simulink model "Teleoperation_Config_Space"  (R2021b)
settings: Solver=FixedStepAuto  StartTime=0.0  StopTime=4  FixedStep=Ts  RelTol=1e-3
values from neighbouring files (symbols this model uses):
  alphas_m = 75.0 * ones(1,n)    [setup_teleop.m]
  B_m = diag(ones(1,n)) * 5    [setup_teleop.m]
  B_s = diag(ones(1,n)) * 4    [setup_teleop.m]
  G = 15    [setup_teleop.m]
  gravity = [0 0 9.81]'    [setup_robot.m]
  K_g = eye(n) * k_g    [setup_teleop.m]
  K_m = diag(ones(1,n)) * 10    [setup_teleop.m]
  K_s = diag(ones(1,n)) * 4    [setup_teleop.m]
  lambdas_m = 4.0 * ones(1,n)    [setup_teleop.m]
  M_m = diag(ones(1,n)) * 1    [setup_teleop.m]
  M_s = diag(ones(1,n)) * 1    [setup_teleop.m]
  T_m2s = 0    [setup_teleop.m]
  T_s2m = 0    [setup_teleop.m]
  zdq_A = [1 3*wc 3*wc^2 wc^3]    [setup_teleop.m]
  zdq_B = [0 0 0 wc^3]    [setup_teleop.m]
undefined symbols (not defined in the file or in its folder): alphas_s, conf, dh, Fm_A, Fm_B, Fs_A, Fs_B, lambdas_s, x0
libraries: vrlib x2, simulink x1
settings Model: Creator=eros  LastModifiedBy=Sebastiano
settings SolverCC: AlgebraicLoopSolver=TrustRegion
settings DebuggingCC: SFMachineParentedDataDiag=warning

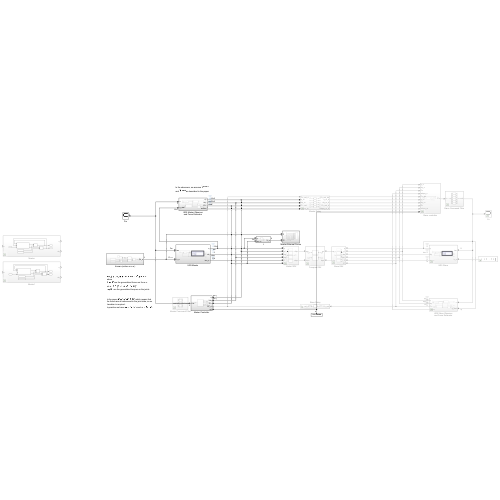
[thumbnail: Simulink's stored preview of the top-level diagram]
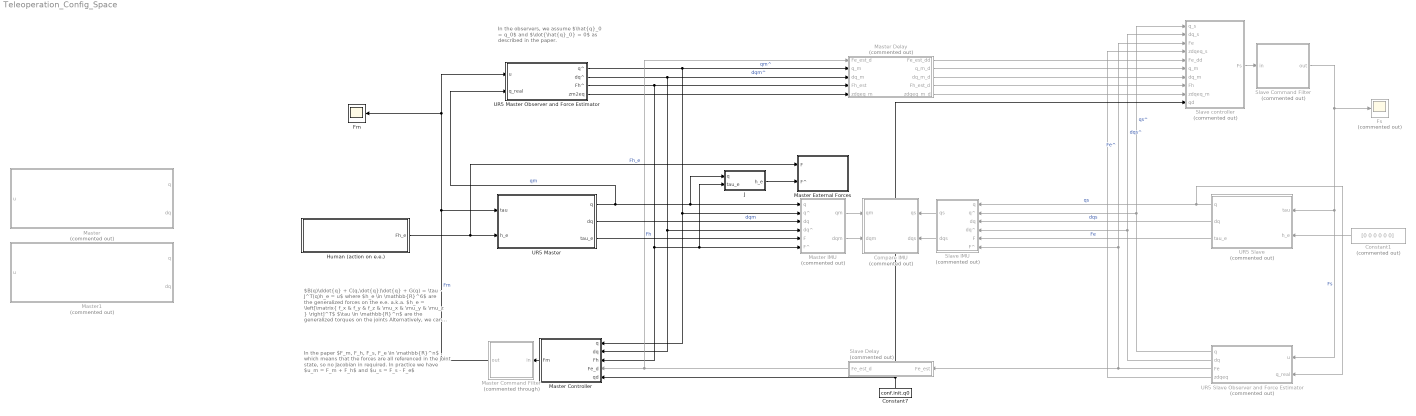
== system Teleoperation_Config_Space ==
  note: In the observers, we assume $\hat{q}_0 = q_0$ and $\dot{\hat{q}_0} = 0$ as described in the paper.
  note: In the paper $F_m, F_h, F_s, F_e \in \mathbb{R}^n$ , which means that the forces are all referenced in the joint state, so no Jacobian in required.
      | In practice we have $u_m = F_m + F_h$ and $u_s = F_s - F_e$
  note: $B(q)\ddot{q} + C(q,\dot{q})\dot{q} + G(q) = \tau - J^T(q)h_e = u$
      | where
      | $h_e \in \mathbb{R}^6$ are the generalized forces on the e.e.
      | a.k.a. $h_e = \left[\matrix{ f_x & f_y & f_z & \mu_x & \mu_y & \mu_z } \right]^T$
      | $\tau \in \mathbb{R}^n$ are the generalized torques on the joints
      |
      | Alternatively, we can write $\tau = J^T(q)\tau_e$ .
  Compare IMU : Subsystem  Commented=on
      settings: PortSchema="{\"entries\":[{\"content\":{\"sides\":[{\"content\":{\"connectorIds\":[\"In1\",\"In2\"]},\"type\":\"ConnectorPlacement.EquallySpacedRectSide\",\"uuid\":\"eee4eb85-6cb8-4462-85fc-1aafb3c3937f\"},{\"content\":{\"connectorIds\":[\"In3\",\"In4\"],\"side\":\"RIGHT\"},\"type\":\"ConnectorPlacement.EquallySpacedRectSide\",\"uuid\":\"5ab37ec6-6ee1-47e9-aff6-41baaee9b59b\"},{\"content\":{\"connectorIds\":[],\"side\":\"TOP\"},\"type\":\"ConnectorPlacement.EquallySpacedRectSide\",\"uuid\":\"6f11ee79-2d90-4b50-8360-b99d360f33b3\"}]},\"type\":\"ConnectorPlacement.EquallySpacedConnector\",\"uuid\":\"5676dc65-12f4-4a54-a0ce-a07c6c462ad2\"}],\"packageUris\":[\"http://schema.mathworks.com/mf0/Connector/R2020b\"],\"version\":\"1.0\"}"
  Constant1 : Constant  Commented=on  Value=[0 0 0 0 0 0]
  Constant7 : Constant  Value=conf.init.q0
  Fm : Scope
  Fs : Scope  Commented=on
  Human (action on e.e.) : Subsystem
  J : Subsystem
  Master : Subsystem  Commented=on
  Master Command Filter : Subsystem  Commented=through
  Master Controller : Subsystem
  Master Delay : Subsystem  Commented=on
  Master External Forces : Subsystem
  Master IMU : Subsystem  Commented=on
  Master1 : Subsystem  Commented=on
  Slave Command Filter : Subsystem  Commented=on
  Slave Delay : Subsystem  Commented=on
  Slave IMU : Subsystem  Commented=on
  Slave controller : Subsystem  Commented=on
  UR5 Master : Subsystem
  UR5 Master Observer and Force Estimator : Subsystem
  UR5 Slave : Subsystem  Commented=on
  UR5 Slave Observer and Force Estimator : Subsystem  Commented=on
  wires:
  UR5 Slave Observer and Force Estimator/1(q) -> Slave IMU/2(q^), Slave controller/1(q_s)  "qs^"
  Master Controller/1(Fm) -> Master Command Filter/1(in)
  UR5 Slave Observer and Force Estimator/4(zdqeq) -> Slave controller/4(zdqeq_s)
  UR5 Master Observer and Force Estimator/1(q^) -> Master Controller/1(q), Master IMU/2(q^), Master Delay/2(q_m)  "qm^"
  UR5 Slave Observer and Force Estimator/3(Fe) -> Slave controller/3(Fe), Slave IMU/6(F^), Slave Delay/1(Fe_est)  "Fe^"
  UR5 Master Observer and Force Estimator/3(Fh^) -> Master IMU/6(F^), J/2(tau_e), Master Controller/3(Fh), Master Delay/4(Fh_est)
  UR5 Slave Observer and Force Estimator/2(dq) -> Slave IMU/4(dq^), Slave controller/2(dq_s)  "dqs^"
  UR5 Master Observer and Force Estimator/2(dq^) -> Master Controller/2(dq), Master IMU/4(dq^), Master Delay/3(dq_m)  "dqm^"
  Slave controller/1(Fs) -> Slave Command Filter/1(in)
  Master Command Filter/1(out) -> UR5 Master Observer and Force Estimator/1(u), Fm/1, UR5 Master/1(tau)  "Fm"
  Slave Command Filter/1(out) -> UR5 Slave/1(tau), UR5 Slave Observer and Force Estimator/1(u), Fs/1  "Fs"
  UR5 Master Observer and Force Estimator/4(zm2eq) -> Master Delay/5(zdqeq_m)
  Master Delay/1(Fe_est_dd) -> Slave controller/5(Fe_dd)
  Master Delay/3(dq_m_d) -> Slave controller/7(dq_m)
  Master Delay/2(q_m_d) -> Slave controller/6(q_m)
  Master Delay/4(Fh_est_d) -> Slave controller/8(Fh)
  Master Delay/5(zdqeq_m_d) -> Slave controller/9(zdqeq_m)
  Slave Delay/1(Fe_est_d) -> Master Delay/1(Fe_est_d), Master Controller/4(Fe_d)
  UR5 Slave/1(q) -> UR5 Slave Observer and Force Estimator/2(q_real), Slave IMU/1(q)  "qs"
  UR5 Slave/2(dq) -> Slave IMU/3(dq)  "dqs"
  Constant1/1 -> UR5 Slave/2(h_e)
  UR5 Slave/3(tau_e) -> Slave IMU/5(F)  "Fe"
  Constant7/1 -> Master Controller/5(qd), Slave controller/10(qd)
  J/1(h_e) -> Master External Forces/2(F^)
  Human (action on e.e.)/1(Fh_e) -> Master External Forces/1(F), UR5 Master/2(h_e)  "Fh_e"
  UR5 Master/1(q) -> UR5 Master Observer and Force Estimator/2(q_real), J/1(q), Master IMU/1(q)  "qm"
  UR5 Master/2(dq) -> Master IMU/3(dq)  "dqm"
  UR5 Master/3(tau_e) -> Master IMU/5(F)  "Fh"
  Master IMU/1(qm) -> Compare IMU/1(qm)
  Master IMU/2(dqm) -> Compare IMU/2(dqm)
  Slave IMU/1(qs) -> Compare IMU/3(qs)
  Slave IMU/2(dqs) -> Compare IMU/4(dqs)

== system Teleoperation_Config_Space/Compare IMU ==
  qm : Inport
  dqm : Inport  Port=2
  qs : Inport  Port=3
  dqs : Inport  Port=4
  State : Subsystem
      settings: PortSchema="{\"entries\":[{\"content\":{\"sides\":[{\"content\":{\"connectorIds\":[\"In1\"]},\"type\":\"ConnectorPlacement.EquallySpacedRectSide\",\"uuid\":\"98f8c5d8-e26e-427c-a81e-60bbe3a3ab4d\"},{\"content\":{\"connectorIds\":[\"In2\"],\"side\":\"RIGHT\"},\"type\":\"ConnectorPlacement.EquallySpacedRectSide\",\"uuid\":\"a51aa647-09cd-4fb3-b31a-f2bc2bc6e0ff\"},{\"content\":{\"connectorIds\":[],\"side\":\"TOP\"},\"type\":\"ConnectorPlacement.EquallySpacedRectSide\",\"uuid\":\"9387bbe5-2fda-43cb-b346-55f243092f42\"}]},\"type\":\"ConnectorPlacement.EquallySpacedConnector\",\"uuid\":\"8debe184-3b59-4f16-84f4-2d6030e17ba5\"}],\"packageUris\":[\"http://schema.mathworks.com/mf0/Connector/R2020b\"],\"version\":\"1.0\"}"
  Velocity : Subsystem
      settings: PortSchema="{\"entries\":[{\"content\":{\"sides\":[{\"content\":{\"connectorIds\":[\"In1\"]},\"type\":\"ConnectorPlacement.EquallySpacedRectSide\",\"uuid\":\"98f8c5d8-e26e-427c-a81e-60bbe3a3ab4d\"},{\"content\":{\"connectorIds\":[\"In2\"],\"side\":\"RIGHT\"},\"type\":\"ConnectorPlacement.EquallySpacedRectSide\",\"uuid\":\"a51aa647-09cd-4fb3-b31a-f2bc2bc6e0ff\"},{\"content\":{\"connectorIds\":[],\"side\":\"TOP\"},\"type\":\"ConnectorPlacement.EquallySpacedRectSide\",\"uuid\":\"9387bbe5-2fda-43cb-b346-55f243092f42\"}]},\"type\":\"ConnectorPlacement.EquallySpacedConnector\",\"uuid\":\"8debe184-3b59-4f16-84f4-2d6030e17ba5\"}],\"packageUris\":[\"http://schema.mathworks.com/mf0/Connector/R2020b\"],\"version\":\"1.0\"}"
  wires:
  qm/1 -> State/2(q_m)
  qs/1 -> State/1(q_s)
  dqm/1 -> Velocity/1(dq_m)
  dqs/1 -> Velocity/2(dq_s)

== system Teleoperation_Config_Space/Human (action on e.e.) ==
  Constant2 : Constant  Value=[0 1 0 0 0 0]
  Constant4 : Constant  Value=[0 0 1 0 0 0]
  Manual Switch : ManualSwitch  CurrentSetting=0
  Matrix Multiply : Product
  Multiply : Gain  Gain=G
  Pulse Generator : DiscretePulseGenerator  PulseType=Time based  TimeSource=Use external signal  Period=1.5  PulseWidth=50  PhaseDelay=0.5
  Switch : Switch  Criteria=u2 > Threshold  Threshold=1.75
  Time : simulink/Sources/Ramp  slope=1  start=0  InitialOutput=0
  Transfer Fcn : TransferFcn  Numerator=[2*pi*5]  Denominator=[1 2*pi*5]
  Fh_e : Outport
  wires:
  Pulse Generator/1 -> Multiply/1
  Switch/1 -> Matrix Multiply/2
  Constant2/1 -> Manual Switch/2
  Transfer Fcn/1 -> Matrix Multiply/1
  Time/1 -> Switch/2, Pulse Generator/1
  Constant4/1 -> Manual Switch/1, Switch/1
  Matrix Multiply/1 -> Fh_e/1
  Multiply/1 -> Transfer Fcn/1
  Manual Switch/1 -> Switch/3

== system Teleoperation_Config_Space/J ==
  q : Inport
  tau_e : Inport  Port=2
  MATLAB Function : MATLAB Function  TreatAsAtomicUnit=on
  Matrix Multiply : Product  Multiplication=Matrix(*)
  h_e : Outport
  wires:
  MATLAB Function/1(J) -> Matrix Multiply/1
  Matrix Multiply/1 -> h_e/1
  tau_e/1 -> Matrix Multiply/2
  q/1 -> MATLAB Function/1(q)

== system Teleoperation_Config_Space/Master ==
  u : Inport
  Constant : Constant  Value=conf.init.q0
  Constant1 : Constant  Value=conf.init.dq0
  Integrator : Integrator  InitialConditionSource=external
  Integrator1 : Integrator  InitialConditionSource=external
  MATLAB Function : MATLAB Function  TreatAsAtomicUnit=on
  q : Outport
  dq : Outport  Port=2
  wires:
  MATLAB Function/1(dq) -> Integrator/1
  MATLAB Function/2(ddq) -> Integrator1/1
  Integrator/1 -> MATLAB Function/1(q), q/1
  Integrator1/1 -> MATLAB Function/2("dq "), dq/1
  u/1 -> MATLAB Function/3(u)
  Constant/1 -> Integrator/2
  Constant1/1 -> Integrator1/2

== system Teleoperation_Config_Space/Master Command Filter ==
  in : Inport
  Demux : Demux  Outputs=6
  Filter{,1..5} (6 alike) : TransferFcn  Numerator=Fm_B  Denominator=Fm_A
  Mux : Mux  Inputs=6
  out : Outport
  wires:
  Demux/4 -> Filter3/1
  Demux/6 -> Filter5/1
  Demux/2 -> Filter1/1
  Demux/5 -> Filter4/1
  Demux/1 -> Filter/1
  Demux/3 -> Filter2/1
  in/1 -> Demux/1
  Mux/1 -> out/1
  Filter/1 -> Mux/1
  Filter1/1 -> Mux/2
  Filter2/1 -> Mux/3
  Filter3/1 -> Mux/4
  Filter4/1 -> Mux/5
  Filter5/1 -> Mux/6

== system Teleoperation_Config_Space/Master Controller ==
  q : Inport
  dq : Inport  Port=2
  Fh : Inport  Port=3
  Fe_d : Inport  Port=4
  qd : Inport  Port=5
  Master Controller : MATLAB Function  TreatAsAtomicUnit=on
  Fm : Outport
  wires:
  Fh/1 -> Master Controller/3(Fh)
  Fe_d/1 -> Master Controller/4(Fe_d)
  Master Controller/1(Fm) -> Fm/1  "Fm"
  q/1 -> Master Controller/1(q)
  dq/1 -> Master Controller/2(dq)
  qd/1 -> Master Controller/5(qd)

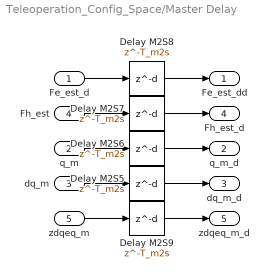
== system Teleoperation_Config_Space/Master Delay ==
  Fe_est_d : Inport
  q_m : Inport  Port=2
  dq_m : Inport  Port=3
  Fh_est : Inport  Port=4
  zdqeq_m : Inport  Port=5
  Delay M2S{5..9} (5 alike) : Delay  DelayLength=T_m2s
  Fe_est_dd : Outport
  q_m_d : Outport  Port=2
  dq_m_d : Outport  Port=3
  Fh_est_d : Outport  Port=4
  zdqeq_m_d : Outport  Port=5
  wires:
  zdqeq_m/1 -> Delay M2S9/1
  Delay M2S6/1 -> q_m_d/1
  dq_m/1 -> Delay M2S5/1
  Fe_est_d/1 -> Delay M2S8/1
  Fh_est/1 -> Delay M2S7/1
  Delay M2S5/1 -> dq_m_d/1
  Delay M2S7/1 -> Fh_est_d/1
  q_m/1 -> Delay M2S6/1
  Delay M2S8/1 -> Fe_est_dd/1
  Delay M2S9/1 -> zdqeq_m_d/1

== system Teleoperation_Config_Space/Master External Forces ==
  F : Inport
  F^ : Inport  Port=2
  Master he : Scope  NumInputPorts=6
  Mux{,1..2,4..6} (6 alike) : Mux  Inputs=2
  qm : Demux  Outputs=dh.dof
  qs : Demux  Outputs=dh.dof
  wires:
  F/1 -> qm/1
  F^/1 -> qs/1
  qm/1 -> Mux/1
  qs/1 -> Mux/2
  qm/2 -> Mux1/1
  qs/2 -> Mux1/2
  qm/3 -> Mux2/1
  qs/3 -> Mux2/2
  qm/4 -> Mux4/1
  qs/4 -> Mux4/2
  Mux/1 -> Master he/1
  Mux1/1 -> Master he/2
  Mux2/1 -> Master he/3
  Mux4/1 -> Master he/4
  Mux5/1 -> Master he/5
  Mux6/1 -> Master he/6
  qs/5 -> Mux5/2
  qm/5 -> Mux5/1
  qm/6 -> Mux6/1
  qs/6 -> Mux6/2

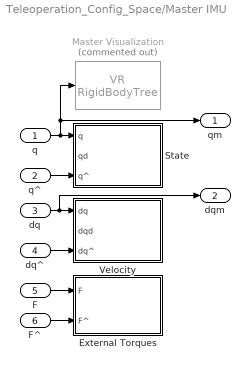
== system Teleoperation_Config_Space/Master IMU ==
  q : Inport
  q^ : Inport  Port=2
  dq : Inport  Port=3
  dq^ : Inport  Port=4
  F : Inport  Port=5
  F^ : Inport  Port=6
  External Torques : Subsystem
  Master Visualization : vrlib/VR RigidBodyTree  Commented=on  RBT=UR5_robot  useRBT=on  Ts=-1  ForceViewerOpen=on
      settings: SourceProductBaseCode=SL
  State : Subsystem
  Velocity : Subsystem
  qm : Outport
  dqm : Outport  Port=2
  wires:
  q/1 -> Master Visualization/1, qm/1, State/1(q)
  q^/1 -> State/3(q^)
  dq/1 -> dqm/1, Velocity/1(dq)
  dq^/1 -> Velocity/3(dq^)
  F/1 -> External Torques/1(F)
  F^/1 -> External Torques/2(F^)

== system Teleoperation_Config_Space/Master1 ==
  u : Inport
  Constant : Constant  Value=conf.init.q0
  Constant1 : Constant  Value=conf.init.dq0
  Integrator : Integrator  InitialConditionSource=external
  Integrator1 : Integrator  InitialConditionSource=external
  MATLAB Function : MATLAB Function  TreatAsAtomicUnit=on
  q : Outport
  dq : Outport  Port=2
  wires:
  MATLAB Function/1(dX) -> Integrator/1
  MATLAB Function/2(ddX) -> Integrator1/1
  Integrator/1 -> q/1, MATLAB Function/1(X)
  Integrator1/1 -> MATLAB Function/2("dX "), dq/1
  u/1 -> MATLAB Function/4(u)
  Constant/1 -> Integrator/2
  Constant1/1 -> Integrator1/2

== system Teleoperation_Config_Space/Slave Command Filter ==
  in : Inport
  Demux : Demux  Outputs=6
  Filter{,1..5} (6 alike) : TransferFcn  Numerator=Fs_B  Denominator=Fs_A
  Mux : Mux  Inputs=6
  out : Outport
  wires:
  Demux/4 -> Filter3/1
  Demux/6 -> Filter5/1
  Demux/2 -> Filter1/1
  Demux/5 -> Filter4/1
  Demux/1 -> Filter/1
  Demux/3 -> Filter2/1
  in/1 -> Demux/1
  Mux/1 -> out/1
  Filter/1 -> Mux/1
  Filter2/1 -> Mux/3
  Filter3/1 -> Mux/4
  Filter4/1 -> Mux/5
  Filter5/1 -> Mux/6
  Filter1/1 -> Mux/2

== system Teleoperation_Config_Space/Slave Delay ==
  Fe_est : Inport
  Delay S2M1 : Delay  DelayLength=T_s2m
  Fe_est_d : Outport
  wires:
  Delay S2M1/1 -> Fe_est_d/1
  Fe_est/1 -> Delay S2M1/1

== system Teleoperation_Config_Space/Slave IMU ==
  q : Inport
  q^ : Inport  Port=2
  dq : Inport  Port=3
  dq^ : Inport  Port=4
  F : Inport  Port=5
  F^ : Inport  Port=6
  External Forces : Subsystem
  Master Visualization : vrlib/VR RigidBodyTree  Commented=on  RBT=UR5_robot  useRBT=on  Ts=-1  ForceViewerOpen=on
      settings: SourceProductBaseCode=SL
  State : Subsystem
  Velocity : Subsystem
  qs : Outport
  dqs : Outport  Port=2
  wires:
  q/1 -> Master Visualization/1, qs/1, State/1(q)
  q^/1 -> State/3(q^)
  F/1 -> External Forces/1(F)
  dq/1 -> dqs/1, Velocity/1(dq)
  F^/1 -> External Forces/2(F^)
  dq^/1 -> Velocity/3(dq^)

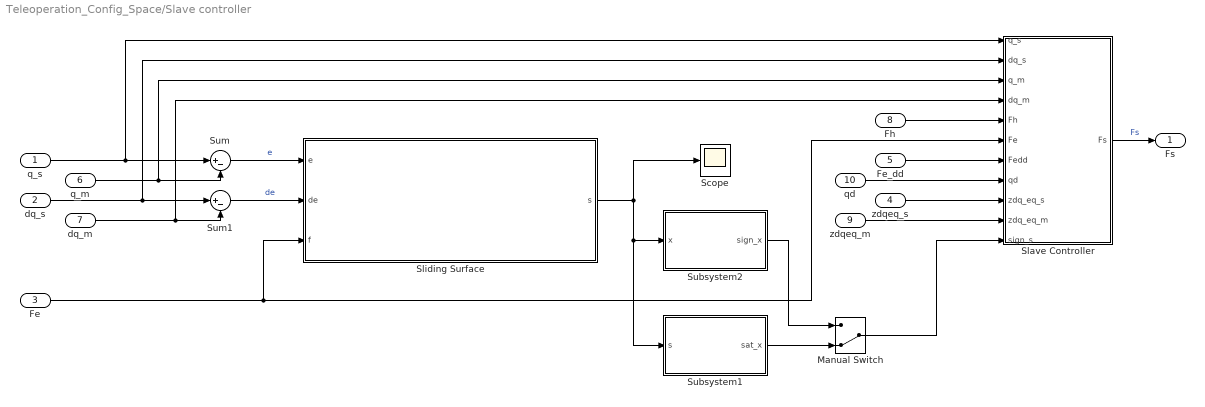
== system Teleoperation_Config_Space/Slave controller ==
  q_s : Inport
  dq_s : Inport  Port=2
  Fe : Inport  Port=3
  zdqeq_s : Inport  Port=4
  Fe_dd : Inport  Port=5
  q_m : Inport  Port=6
  dq_m : Inport  Port=7
  Fh : Inport  Port=8
  zdqeq_m : Inport  Port=9
  qd : Inport  Port=10
  Manual Switch : ManualSwitch  CurrentSetting=0
  Scope : Scope
  Slave Controller : MATLAB Function  TreatAsAtomicUnit=on
  Sliding Surface : Subsystem
  Subsystem1 : Subsystem
  Subsystem2 : Subsystem
  Sum : Sum  Inputs=|+-
  Sum1 : Sum  Inputs=|+-
  Fs : Outport
  wires:
  zdqeq_s/1 -> Slave Controller/9(zdq_eq_s)
  Fh/1 -> Slave Controller/5(Fh)
  Slave Controller/1(Fs) -> Fs/1  "Fs"
  zdqeq_m/1 -> Slave Controller/10(zdq_eq_m)
  Fe_dd/1 -> Slave Controller/7(Fedd)
  q_s/1 -> Sum/1, Slave Controller/1(q_s)
  q_m/1 -> Sum/2, Slave Controller/3(q_m)
  dq_s/1 -> Sum1/1, Slave Controller/2(dq_s)
  dq_m/1 -> Slave Controller/4(dq_m), Sum1/2
  Fe/1 -> Slave Controller/6(Fe), Sliding Surface/3(f)
  Subsystem2/1(sign_x) -> Manual Switch/1
  Sum/1 -> Sliding Surface/1(e)  "e"
  Sum1/1 -> Sliding Surface/2(de)  "de"
  Sliding Surface/1(s) -> Scope/1, Subsystem1/1(s), Subsystem2/1(x)
  qd/1 -> Slave Controller/8(qd)
  Subsystem1/1(sat_x) -> Manual Switch/2
  Manual Switch/1 -> Slave Controller/11(sign_s)

== system Teleoperation_Config_Space/UR5 Master ==
  note: UR5
  tau : Inport
  h_e : Inport  Port=2
  Constant2 : Constant  Value=conf.init.dq0
  Constant6 : Constant  Value=gravity
  Constant7 : Constant  Value=conf.init.q0
  JT : Subsystem
  Robot Model : Subsystem
  Sum4 : Sum  Inputs=++|
  q : Outport
  dq : Outport  Port=2
  tau_e : Outport  Port=3
  wires:
  Robot Model/1(dq) -> dq/1
  tau/1 -> Sum4/1
  Robot Model/2(q) -> JT/2(q), q/1
  JT/1(tau_e) -> tau_e/1, Sum4/2
  h_e/1 -> JT/1(h_e)
  Constant7/1 -> Robot Model/4(q0)
  Constant2/1 -> Robot Model/3(dq0)
  Constant6/1 -> Robot Model/2(g)
  Sum4/1 -> Robot Model/1(u)

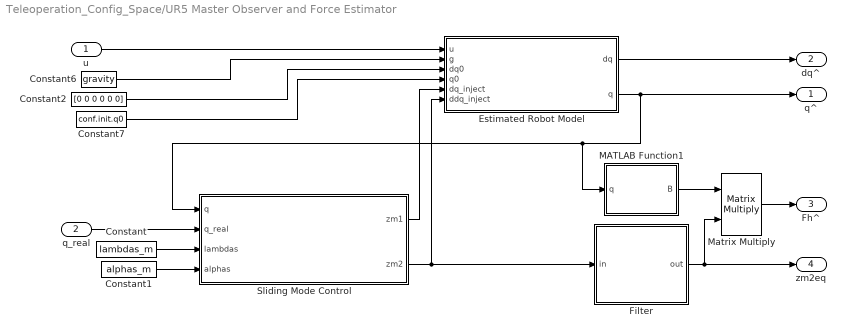
== system Teleoperation_Config_Space/UR5 Master Observer and Force Estimator ==
  u : Inport
  q_real : Inport  Port=2
  Constant : Constant  Value=lambdas_m
  Constant1 : Constant  Value=alphas_m
  Constant2 : Constant  Value=[0 0 0 0 0 0]
  Constant6 : Constant  Value=gravity
  Constant7 : Constant  Value=conf.init.q0
  Estimated Robot Model : Subsystem
  Filter : Subsystem
  MATLAB Function1 : MATLAB Function  TreatAsAtomicUnit=on
  Matrix Multiply : Product  Multiplication=Matrix(*)
  Sliding Mode Control : Subsystem
  q^ : Outport
  dq^ : Outport  Port=2
  Fh^ : Outport  Port=3
  zm2eq : Outport  Port=4
  wires:
  Matrix Multiply/1 -> Fh^/1
  Filter/1(out) -> zm2eq/1, Matrix Multiply/2
  Sliding Mode Control/1(zm1) -> Estimated Robot Model/5(dq_inject)
  Constant7/1 -> Estimated Robot Model/4(q0)
  Constant2/1 -> Estimated Robot Model/3(dq0)
  Constant6/1 -> Estimated Robot Model/2(g)
  u/1 -> Estimated Robot Model/1(u)
  Sliding Mode Control/2(zm2) -> Estimated Robot Model/6(ddq_inject), Filter/1(in)
  MATLAB Function1/1(B) -> Matrix Multiply/1
  Constant1/1 -> Sliding Mode Control/4(alphas)
  Constant/1 -> Sliding Mode Control/3(lambdas)
  q_real/1 -> Sliding Mode Control/2(q_real)
  Estimated Robot Model/2(q) -> q^/1, MATLAB Function1/1(q), Sliding Mode Control/1(q)
  Estimated Robot Model/1(dq) -> dq^/1

== system Teleoperation_Config_Space/UR5 Slave ==
  note: UR5
  tau : Inport
  h_e : Inport  Port=2
  Constant2 : Constant  Value=conf.init.dq0
  Constant6 : Constant  Value=gravity
  Constant7 : Constant  Value=conf.init.q0
  JT : Subsystem
  Robot Model : Subsystem
  Sum4 : Sum  Inputs=+-|
  q : Outport
  dq : Outport  Port=2
  tau_e : Outport  Port=3
  wires:
  Robot Model/1(dq) -> dq/1
  tau/1 -> Sum4/1
  Robot Model/2(q) -> JT/2(q), q/1
  JT/1(tau_e) -> tau_e/1, Sum4/2
  h_e/1 -> JT/1(h_e)
  Constant7/1 -> Robot Model/4(q0)
  Constant2/1 -> Robot Model/3(dq0)
  Constant6/1 -> Robot Model/2(g)
  Sum4/1 -> Robot Model/1(u)

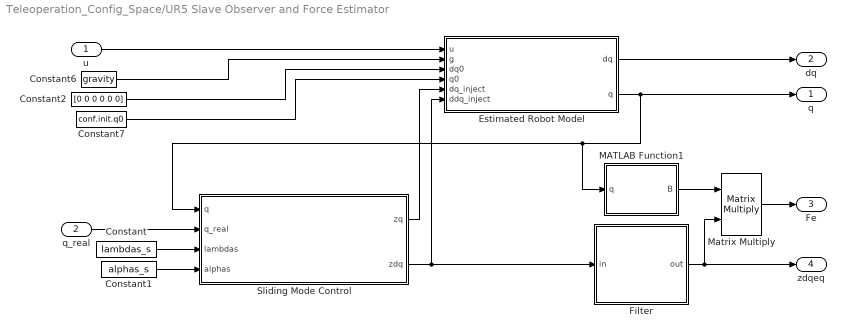
== system Teleoperation_Config_Space/UR5 Slave Observer and Force Estimator ==
  u : Inport
  q_real : Inport  Port=2
  Constant : Constant  Value=lambdas_s
  Constant1 : Constant  Value=alphas_s
  Constant2 : Constant  Value=[0 0 0 0 0 0]
  Constant6 : Constant  Value=gravity
  Constant7 : Constant  Value=conf.init.q0
  Estimated Robot Model : Subsystem
  Filter : Subsystem
  MATLAB Function1 : MATLAB Function  TreatAsAtomicUnit=on
  Matrix Multiply : Product  Multiplication=Matrix(*)
  Sliding Mode Control : Subsystem
  q : Outport
  dq : Outport  Port=2
  Fe : Outport  Port=3
  zdqeq : Outport  Port=4
  wires:
  Estimated Robot Model/2(q) -> MATLAB Function1/1(q), Sliding Mode Control/1(q), q/1
  Estimated Robot Model/1(dq) -> dq/1
  Matrix Multiply/1 -> Fe/1
  Filter/1(out) -> zdqeq/1, Matrix Multiply/2
  Sliding Mode Control/1(zq) -> Estimated Robot Model/5(dq_inject)
  Constant7/1 -> Estimated Robot Model/4(q0)
  Constant2/1 -> Estimated Robot Model/3(dq0)
  Constant6/1 -> Estimated Robot Model/2(g)
  u/1 -> Estimated Robot Model/1(u)
  Sliding Mode Control/2(zdq) -> Filter/1(in), Estimated Robot Model/6(ddq_inject)
  MATLAB Function1/1(B) -> Matrix Multiply/1
  Constant1/1 -> Sliding Mode Control/4(alphas)
  Constant/1 -> Sliding Mode Control/3(lambdas)
  q_real/1 -> Sliding Mode Control/2(q_real)

== system Teleoperation_Config_Space/Compare IMU/State ==
  q_s : Inport
  q_m : Inport  Port=2
  Compare State : Scope  NumInputPorts=6
  Mux{,1..2,4..6} (6 alike) : Mux  Inputs=2
  qm : Demux  Outputs=dh.dof
  qs : Demux  Outputs=dh.dof
  wires:
  q_m/1 -> qm/1
  q_s/1 -> qs/1
  qm/1 -> Mux/1
  qs/1 -> Mux/2
  qm/2 -> Mux1/1
  qs/2 -> Mux1/2
  qm/3 -> Mux2/1
  qs/3 -> Mux2/2
  qm/4 -> Mux4/1
  qs/4 -> Mux4/2
  Mux/1 -> Compare State/1
  Mux1/1 -> Compare State/2
  Mux2/1 -> Compare State/3
  Mux4/1 -> Compare State/4
  Mux5/1 -> Compare State/5
  Mux6/1 -> Compare State/6
  qs/5 -> Mux5/2
  qm/5 -> Mux5/1
  qm/6 -> Mux6/1
  qs/6 -> Mux6/2

== system Teleoperation_Config_Space/Compare IMU/Velocity ==
  dq_m : Inport
  dq_s : Inport  Port=2
  Compare Speed : Scope  NumInputPorts=6
  Mux{,1..2,4..6} (6 alike) : Mux  Inputs=2
  qm : Demux  Outputs=dh.dof
  qs : Demux  Outputs=dh.dof
  wires:
  dq_m/1 -> qm/1
  dq_s/1 -> qs/1
  qm/1 -> Mux/1
  qs/1 -> Mux/2
  qm/2 -> Mux1/1
  qs/2 -> Mux1/2
  qm/3 -> Mux2/1
  qs/3 -> Mux2/2
  qm/4 -> Mux4/1
  qs/4 -> Mux4/2
  Mux/1 -> Compare Speed/1
  Mux1/1 -> Compare Speed/2
  Mux2/1 -> Compare Speed/3
  Mux4/1 -> Compare Speed/4
  Mux5/1 -> Compare Speed/5
  Mux6/1 -> Compare Speed/6
  qs/5 -> Mux5/2
  qm/5 -> Mux5/1
  qm/6 -> Mux6/1
  qs/6 -> Mux6/2

== system Teleoperation_Config_Space/Master IMU/External Torques ==
  F : Inport
  F^ : Inport  Port=2
  Master Fh : Scope  NumInputPorts=6
  Mux{,1..2,4..6} (6 alike) : Mux  Inputs=2
  qm : Demux  Outputs=dh.dof
  qs : Demux  Outputs=dh.dof
  wires:
  F/1 -> qm/1
  F^/1 -> qs/1
  qm/1 -> Mux/1
  qs/1 -> Mux/2
  qm/2 -> Mux1/1
  qs/2 -> Mux1/2
  qm/3 -> Mux2/1
  qs/3 -> Mux2/2
  qm/4 -> Mux4/1
  qs/4 -> Mux4/2
  Mux/1 -> Master Fh/1
  Mux1/1 -> Master Fh/2
  Mux2/1 -> Master Fh/3
  Mux4/1 -> Master Fh/4
  Mux5/1 -> Master Fh/5
  Mux6/1 -> Master Fh/6
  qs/5 -> Mux5/2
  qm/5 -> Mux5/1
  qm/6 -> Mux6/1
  qs/6 -> Mux6/2

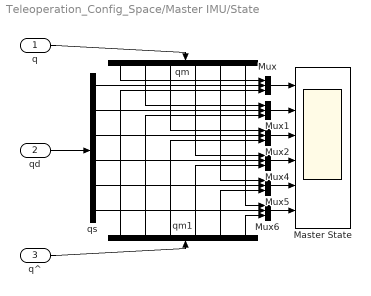
== system Teleoperation_Config_Space/Master IMU/State ==
  q : Inport
  qd : Inport  Port=2
  q^ : Inport  Port=3
  Master State : Scope  NumInputPorts=6
  Mux{,1..2,4..6} (6 alike) : Mux  Inputs=3
  qm : Demux  Outputs=dh.dof
  qm1 : Demux  Outputs=dh.dof
  qs : Demux  Outputs=dh.dof
  wires:
  q/1 -> qm/1
  qd/1 -> qs/1
  qm/1 -> Mux/1
  qs/1 -> Mux/2
  qm/2 -> Mux1/1
  qs/2 -> Mux1/2
  qm/3 -> Mux2/1
  qs/3 -> Mux2/2
  qm/4 -> Mux4/1
  qs/4 -> Mux4/2
  Mux/1 -> Master State/1
  Mux1/1 -> Master State/2
  Mux2/1 -> Master State/3
  Mux4/1 -> Master State/4
  Mux5/1 -> Master State/5
  Mux6/1 -> Master State/6
  qs/5 -> Mux5/2
  qm/5 -> Mux5/1
  qm/6 -> Mux6/1
  qs/6 -> Mux6/2
  qm1/3 -> Mux2/3
  qm1/2 -> Mux1/3
  qm1/4 -> Mux4/3
  qm1/5 -> Mux5/3
  q^/1 -> qm1/1
  qm1/1 -> Mux/3
  qm1/6 -> Mux6/3

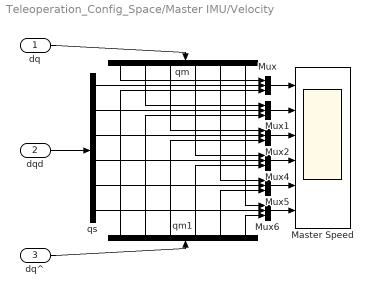
== system Teleoperation_Config_Space/Master IMU/Velocity ==
  dq : Inport
  dqd : Inport  Port=2
  dq^ : Inport  Port=3
  Master Speed : Scope  NumInputPorts=6
  Mux{,1..2,4..6} (6 alike) : Mux  Inputs=3
  qm : Demux  Outputs=dh.dof
  qm1 : Demux  Outputs=dh.dof
  qs : Demux  Outputs=dh.dof
  wires:
  dq/1 -> qm/1
  dqd/1 -> qs/1
  qm/1 -> Mux/1
  qs/1 -> Mux/2
  qm/2 -> Mux1/1
  qs/2 -> Mux1/2
  qm/3 -> Mux2/1
  qs/3 -> Mux2/2
  qm/4 -> Mux4/1
  qs/4 -> Mux4/2
  Mux/1 -> Master Speed/1
  Mux1/1 -> Master Speed/2
  Mux2/1 -> Master Speed/3
  Mux4/1 -> Master Speed/4
  Mux5/1 -> Master Speed/5
  Mux6/1 -> Master Speed/6
  qs/5 -> Mux5/2
  qm/5 -> Mux5/1
  qm/6 -> Mux6/1
  qs/6 -> Mux6/2
  qm1/3 -> Mux2/3
  qm1/2 -> Mux1/3
  qm1/4 -> Mux4/3
  qm1/5 -> Mux5/3
  dq^/1 -> qm1/1
  qm1/1 -> Mux/3
  qm1/6 -> Mux6/3

== system Teleoperation_Config_Space/Slave IMU/External Forces ==
  F : Inport
  F^ : Inport  Port=2
  Mux{,1..2,4..6} (6 alike) : Mux  Inputs=2
  Slave Fe : Scope  NumInputPorts=6
  qm : Demux  Outputs=dh.dof
  qs : Demux  Outputs=dh.dof
  wires:
  F/1 -> qm/1
  F^/1 -> qs/1
  qm/1 -> Mux/1
  qs/1 -> Mux/2
  qm/2 -> Mux1/1
  qs/2 -> Mux1/2
  qm/3 -> Mux2/1
  qs/3 -> Mux2/2
  qm/4 -> Mux4/1
  qs/4 -> Mux4/2
  Mux/1 -> Slave Fe/1
  Mux1/1 -> Slave Fe/2
  Mux2/1 -> Slave Fe/3
  Mux4/1 -> Slave Fe/4
  Mux5/1 -> Slave Fe/5
  Mux6/1 -> Slave Fe/6
  qs/5 -> Mux5/2
  qm/5 -> Mux5/1
  qm/6 -> Mux6/1
  qs/6 -> Mux6/2

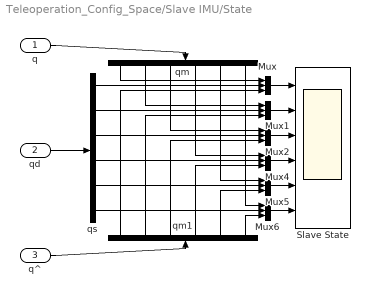
== system Teleoperation_Config_Space/Slave IMU/State ==
  q : Inport
  qd : Inport  Port=2
  q^ : Inport  Port=3
  Mux{,1..2,4..6} (6 alike) : Mux  Inputs=3
  Slave State : Scope  NumInputPorts=6
  qm : Demux  Outputs=dh.dof
  qm1 : Demux  Outputs=dh.dof
  qs : Demux  Outputs=dh.dof
  wires:
  q/1 -> qm/1
  qd/1 -> qs/1
  qm/1 -> Mux/1
  qs/1 -> Mux/2
  qm/2 -> Mux1/1
  qs/2 -> Mux1/2
  qm/3 -> Mux2/1
  qs/3 -> Mux2/2
  qm/4 -> Mux4/1
  qs/4 -> Mux4/2
  Mux/1 -> Slave State/1
  Mux1/1 -> Slave State/2
  Mux2/1 -> Slave State/3
  Mux4/1 -> Slave State/4
  Mux5/1 -> Slave State/5
  Mux6/1 -> Slave State/6
  qs/5 -> Mux5/2
  qm/5 -> Mux5/1
  qm/6 -> Mux6/1
  qs/6 -> Mux6/2
  qm1/3 -> Mux2/3
  qm1/2 -> Mux1/3
  qm1/4 -> Mux4/3
  qm1/5 -> Mux5/3
  q^/1 -> qm1/1
  qm1/1 -> Mux/3
  qm1/6 -> Mux6/3

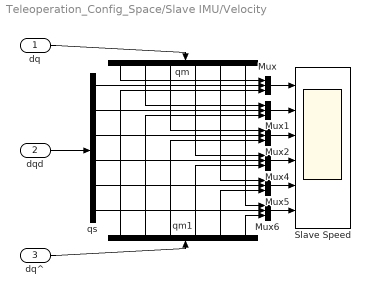
== system Teleoperation_Config_Space/Slave IMU/Velocity ==
  dq : Inport
  dqd : Inport  Port=2
  dq^ : Inport  Port=3
  Mux{,1..2,4..6} (6 alike) : Mux  Inputs=3
  Slave Speed : Scope  NumInputPorts=6
  qm : Demux  Outputs=dh.dof
  qm1 : Demux  Outputs=dh.dof
  qs : Demux  Outputs=dh.dof
  wires:
  dq/1 -> qm/1
  dqd/1 -> qs/1
  qm/1 -> Mux/1
  qs/1 -> Mux/2
  qm/2 -> Mux1/1
  qs/2 -> Mux1/2
  qm/3 -> Mux2/1
  qs/3 -> Mux2/2
  qm/4 -> Mux4/1
  qs/4 -> Mux4/2
  Mux/1 -> Slave Speed/1
  Mux1/1 -> Slave Speed/2
  Mux2/1 -> Slave Speed/3
  Mux4/1 -> Slave Speed/4
  Mux5/1 -> Slave Speed/5
  Mux6/1 -> Slave Speed/6
  qs/5 -> Mux5/2
  qm/5 -> Mux5/1
  qm/6 -> Mux6/1
  qs/6 -> Mux6/2
  qm1/3 -> Mux2/3
  qm1/2 -> Mux1/3
  qm1/4 -> Mux4/3
  qm1/5 -> Mux5/3
  dq^/1 -> qm1/1
  qm1/1 -> Mux/3
  qm1/6 -> Mux6/3

== system Teleoperation_Config_Space/Slave controller/Sliding Surface ==
  e : Inport
  de : Inport  Port=2
  f : Inport  Port=3
  Impedance Model : Subsystem
  Integrator : Integrator
  Multiply3 : Gain  Gain=inv(M_s)  Multiplication=Matrix(K*u)
  s : Outport
  wires:
  Multiply3/1 -> Integrator/1
  e/1 -> Impedance Model/1(e)
  de/1 -> Impedance Model/2(de)
  Integrator/1 -> s/1
  Impedance Model/1(Out1) -> Multiply3/1
  f/1 -> Impedance Model/3(f)

== system Teleoperation_Config_Space/Slave controller/Subsystem1 ==
  s : Inport
  Abs : Abs
  Constant : Constant  Value=10e-2
  Divide : Product  Inputs=*/
  Subsystem2 : Subsystem
  Switch : Switch  Criteria=u2 > Threshold  Threshold=1
  sat_x : Outport
  wires:
  Divide/1 -> Switch/3, Abs/1, Subsystem2/1(x)
  s/1 -> Divide/1
  Constant/1 -> Divide/2
  Abs/1 -> Switch/2
  Switch/1 -> sat_x/1
  Subsystem2/1(sign_x) -> Switch/1

== system Teleoperation_Config_Space/Slave controller/Subsystem2 ==
  x : Inport
  Multiply : Gain  Gain=-1
  Subsystem : Subsystem
  Subsystem1 : Subsystem
  Sum1 : Sum  Inputs=|+-
  sign_x : Outport
  wires:
  Multiply/1 -> Subsystem1/1(In1)
  Subsystem/1(Out1) -> Sum1/1
  Sum1/1 -> sign_x/1
  Subsystem1/1(Out1) -> Sum1/2
  x/1 -> Subsystem/1(In1), Multiply/1

== system Teleoperation_Config_Space/UR5 Master/JT ==
  h_e : Inport
  q : Inport  Port=2
  MATLAB Function : MATLAB Function  TreatAsAtomicUnit=on
  Matrix Multiply : Product  Multiplication=Matrix(*)
  tau_e : Outport
  wires:
  MATLAB Function/1(JT) -> Matrix Multiply/1
  Matrix Multiply/1 -> tau_e/1
  h_e/1 -> Matrix Multiply/2
  q/1 -> MATLAB Function/1(q)

== system Teleoperation_Config_Space/UR5 Master/Robot Model ==
  u : Inport
  g : Inport  Port=2
  dq0 : Inport  Port=3
  q0 : Inport  Port=4
  Integrator : Integrator  InitialConditionSource=external  InitialCondition=x0
  Integrator1 : Integrator  InitialConditionSource=external  InitialCondition=x0
  MATLAB Function : MATLAB Function  TreatAsAtomicUnit=on
  dq : Outport
  q : Outport  Port=2
  wires:
  g/1 -> MATLAB Function/4(g)
  MATLAB Function/1(ddq_) -> Integrator/1
  Integrator1/1 -> q/1, MATLAB Function/2(q)
  u/1 -> MATLAB Function/3(u)
  Integrator/1 -> dq/1, MATLAB Function/1(dq)
  q0/1 -> Integrator1/2
  MATLAB Function/2(dq_) -> Integrator1/1
  dq0/1 -> Integrator/2

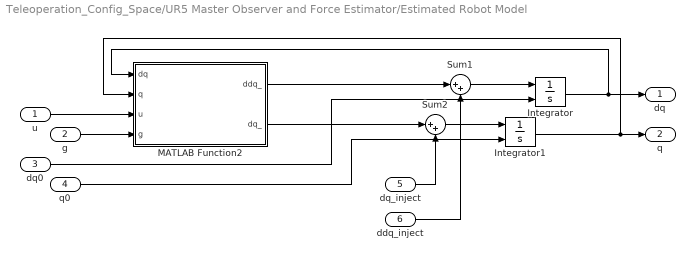
== system Teleoperation_Config_Space/UR5 Master Observer and Force Estimator/Estimated Robot Model ==
  u : Inport
  g : Inport  Port=2
  dq0 : Inport  Port=3
  q0 : Inport  Port=4
  dq_inject : Inport  Port=5
  ddq_inject : Inport  Port=6
  Integrator : Integrator  InitialConditionSource=external  InitialCondition=x0
  Integrator1 : Integrator  InitialConditionSource=external  InitialCondition=x0
  MATLAB Function2 : MATLAB Function  TreatAsAtomicUnit=on
  Sum1 : Sum  Inputs=|++
  Sum2 : Sum  Inputs=|++
  dq : Outport
  q : Outport  Port=2
  wires:
  Sum1/1 -> Integrator/1
  Integrator/1 -> dq/1, MATLAB Function2/1(dq)
  MATLAB Function2/1(ddq_) -> Sum1/1
  MATLAB Function2/2(dq_) -> Sum2/1
  Sum2/1 -> Integrator1/1
  u/1 -> MATLAB Function2/3(u)
  q0/1 -> Integrator1/2
  dq0/1 -> Integrator/2
  g/1 -> MATLAB Function2/4(g)
  dq_inject/1 -> Sum2/2
  ddq_inject/1 -> Sum1/2
  Integrator1/1 -> MATLAB Function2/2(q), q/1

== system Teleoperation_Config_Space/UR5 Master Observer and Force Estimator/Filter ==
  in : Inport
  Demux : Demux  Outputs=6
  Filter{,1..5} (6 alike) : TransferFcn  Numerator=zdq_B  Denominator=zdq_A
  Mux : Mux  Inputs=6
  out : Outport
  wires:
  Demux/4 -> Filter3/1
  Demux/6 -> Filter5/1
  Demux/2 -> Filter1/1
  Demux/5 -> Filter4/1
  Demux/1 -> Filter/1
  Demux/3 -> Filter2/1
  in/1 -> Demux/1
  Mux/1 -> out/1
  Filter/1 -> Mux/1
  Filter1/1 -> Mux/2
  Filter2/1 -> Mux/3
  Filter3/1 -> Mux/4
  Filter4/1 -> Mux/5
  Filter5/1 -> Mux/6

== system Teleoperation_Config_Space/UR5 Master Observer and Force Estimator/Sliding Mode Control ==
  q : Inport
  q_real : Inport  Port=2
  lambdas : Inport  Port=3
  alphas : Inport  Port=4
  Abs : Abs
  Matrix Multiply : Product  Inputs=***
  Matrix Multiply1 : Product
  Sqrt : Sqrt  SaturateOnIntegerOverflow=on
  Subsystem2 : Subsystem
  Sum : Sum  Inputs=-+|
  zm1 : Outport
  zm2 : Outport  Port=2
  wires:
  Sum/1 -> Subsystem2/1(x), Abs/1
  Abs/1 -> Sqrt/1
  q/1 -> Sum/1
  lambdas/1 -> Matrix Multiply/3
  Sqrt/1 -> Matrix Multiply/2
  q_real/1 -> Sum/2
  Matrix Multiply/1 -> zm1/1  "zm1"
  Matrix Multiply1/1 -> zm2/1  "zm2"
  alphas/1 -> Matrix Multiply1/2
  Subsystem2/1(sign_x) -> Matrix Multiply/1, Matrix Multiply1/1

== system Teleoperation_Config_Space/UR5 Slave/JT ==
  h_e : Inport
  q : Inport  Port=2
  MATLAB Function : MATLAB Function  TreatAsAtomicUnit=on
  Matrix Multiply : Product  Multiplication=Matrix(*)
  tau_e : Outport
  wires:
  MATLAB Function/1(JT) -> Matrix Multiply/1
  Matrix Multiply/1 -> tau_e/1
  h_e/1 -> Matrix Multiply/2
  q/1 -> MATLAB Function/1(q)

== system Teleoperation_Config_Space/UR5 Slave/Robot Model ==
  u : Inport
  g : Inport  Port=2
  dq0 : Inport  Port=3
  q0 : Inport  Port=4
  Integrator : Integrator  InitialConditionSource=external  InitialCondition=x0
  Integrator1 : Integrator  InitialConditionSource=external  InitialCondition=x0
  MATLAB Function : MATLAB Function  TreatAsAtomicUnit=on
  dq : Outport
  q : Outport  Port=2
  wires:
  g/1 -> MATLAB Function/4(g)
  MATLAB Function/1(ddq_) -> Integrator/1
  Integrator1/1 -> q/1, MATLAB Function/2(q)
  u/1 -> MATLAB Function/3(u)
  Integrator/1 -> dq/1, MATLAB Function/1(dq)
  q0/1 -> Integrator1/2
  MATLAB Function/2(dq_) -> Integrator1/1
  dq0/1 -> Integrator/2

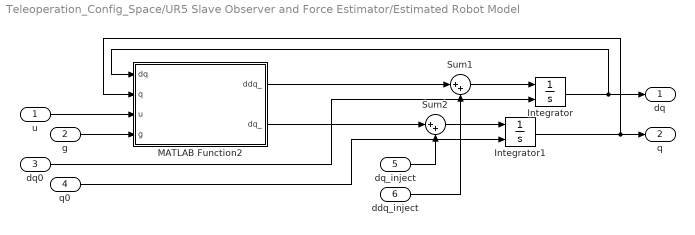
== system Teleoperation_Config_Space/UR5 Slave Observer and Force Estimator/Estimated Robot Model ==
  u : Inport
  g : Inport  Port=2
  dq0 : Inport  Port=3
  q0 : Inport  Port=4
  dq_inject : Inport  Port=5
  ddq_inject : Inport  Port=6
  Integrator : Integrator  InitialConditionSource=external  InitialCondition=x0
  Integrator1 : Integrator  InitialConditionSource=external  InitialCondition=x0
  MATLAB Function2 : MATLAB Function  TreatAsAtomicUnit=on
  Sum1 : Sum  Inputs=|++
  Sum2 : Sum  Inputs=|++
  dq : Outport
  q : Outport  Port=2
  wires:
  Sum1/1 -> Integrator/1
  Integrator/1 -> dq/1, MATLAB Function2/1(dq)
  MATLAB Function2/1(ddq_) -> Sum1/1
  MATLAB Function2/2(dq_) -> Sum2/1
  Sum2/1 -> Integrator1/1
  u/1 -> MATLAB Function2/3(u)
  q0/1 -> Integrator1/2
  dq0/1 -> Integrator/2
  g/1 -> MATLAB Function2/4(g)
  dq_inject/1 -> Sum2/2
  ddq_inject/1 -> Sum1/2
  Integrator1/1 -> MATLAB Function2/2(q), q/1

== system Teleoperation_Config_Space/UR5 Slave Observer and Force Estimator/Filter ==
  in : Inport
  Demux : Demux  Outputs=6
  Filter{,1..5} (6 alike) : TransferFcn  Numerator=zdq_B  Denominator=zdq_A
  Mux : Mux  Inputs=6
  out : Outport
  wires:
  Demux/4 -> Filter3/1
  Demux/6 -> Filter5/1
  Demux/2 -> Filter1/1
  Demux/5 -> Filter4/1
  Demux/1 -> Filter/1
  Demux/3 -> Filter2/1
  in/1 -> Demux/1
  Mux/1 -> out/1
  Filter/1 -> Mux/1
  Filter1/1 -> Mux/2
  Filter2/1 -> Mux/3
  Filter3/1 -> Mux/4
  Filter4/1 -> Mux/5
  Filter5/1 -> Mux/6

== system Teleoperation_Config_Space/UR5 Slave Observer and Force Estimator/Sliding Mode Control ==
  q : Inport
  q_real : Inport  Port=2
  lambdas : Inport  Port=3
  alphas : Inport  Port=4
  Abs : Abs
  Matrix Multiply : Product  Inputs=***
  Matrix Multiply1 : Product
  Sqrt : Sqrt  SaturateOnIntegerOverflow=on
  Subsystem2 : Subsystem
  Sum : Sum  Inputs=-+|
  zq : Outport
  zdq : Outport  Port=2
  wires:
  Sum/1 -> Subsystem2/1(x), Abs/1
  Abs/1 -> Sqrt/1
  q/1 -> Sum/1
  lambdas/1 -> Matrix Multiply/3
  Sqrt/1 -> Matrix Multiply/2
  q_real/1 -> Sum/2
  Matrix Multiply/1 -> zq/1  "zq"
  Matrix Multiply1/1 -> zdq/1  "zdq"
  alphas/1 -> Matrix Multiply1/2
  Subsystem2/1(sign_x) -> Matrix Multiply/1, Matrix Multiply1/1

== system Teleoperation_Config_Space/Slave controller/Sliding Surface/Impedance Model ==
  e : Inport
  de : Inport  Port=2
  f : Inport  Port=3
  Derivative : Derivative  CoefficientInTFapproximation=Ts
  Multiply : Gain  Gain=M_s  Multiplication=Matrix(K*u)
  Multiply1 : Gain  Gain=B_s  Multiplication=Matrix(K*u)
  Multiply2 : Gain  Gain=K_s  Multiplication=Matrix(K*u)
  Sum2 : Sum  Inputs=++++
  Out1 : Outport
  wires:
  Derivative/1 -> Multiply/1  "dde"
  Multiply/1 -> Sum2/3
  Multiply1/1 -> Sum2/2
  de/1 -> Multiply1/1, Derivative/1  "de"
  Multiply2/1 -> Sum2/1
  e/1 -> Multiply2/1  "e"
  f/1 -> Sum2/4
  Sum2/1 -> Out1/1

== system Teleoperation_Config_Space/Slave controller/Subsystem1/Subsystem2 ==
  x : Inport
  Multiply : Gain  Gain=-1
  Subsystem : Subsystem
  Subsystem1 : Subsystem
  Sum1 : Sum  Inputs=|+-
  sign_x : Outport
  wires:
  Multiply/1 -> Subsystem1/1(In1)
  Subsystem/1(Out1) -> Sum1/1
  Sum1/1 -> sign_x/1
  Subsystem1/1(Out1) -> Sum1/2
  x/1 -> Subsystem/1(In1), Multiply/1

== system Teleoperation_Config_Space/Slave controller/Subsystem2/Subsystem ==
  In1 : Inport
  Abs1 : Abs
  Constant : Constant
  Divide : Product  Inputs=*/
  Floor1 : Rounding
  Sum1 : Sum  Inputs=|++
  Out1 : Outport
  wires:
  Divide/1 -> Floor1/1
  Constant/1 -> Sum1/2
  Abs1/1 -> Sum1/1
  In1/1 -> Abs1/1, Divide/1
  Sum1/1 -> Divide/2
  Floor1/1 -> Out1/1

== system Teleoperation_Config_Space/Slave controller/Subsystem2/Subsystem1 ==
  In1 : Inport
  Abs1 : Abs
  Constant : Constant
  Divide : Product  Inputs=*/
  Floor1 : Rounding
  Sum1 : Sum  Inputs=|++
  Out1 : Outport
  wires:
  Divide/1 -> Floor1/1
  Constant/1 -> Sum1/2
  Abs1/1 -> Sum1/1
  In1/1 -> Abs1/1, Divide/1
  Sum1/1 -> Divide/2
  Floor1/1 -> Out1/1

== system Teleoperation_Config_Space/UR5 Master Observer and Force Estimator/Sliding Mode Control/Subsystem2 ==
  x : Inport
  Multiply : Gain  Gain=-1
  Subsystem : Subsystem
  Subsystem1 : Subsystem
  Sum1 : Sum  Inputs=|+-
  sign_x : Outport
  wires:
  Multiply/1 -> Subsystem1/1(In1)
  Subsystem/1(Out1) -> Sum1/1
  Sum1/1 -> sign_x/1
  Subsystem1/1(Out1) -> Sum1/2
  x/1 -> Subsystem/1(In1), Multiply/1

== system Teleoperation_Config_Space/UR5 Slave Observer and Force Estimator/Sliding Mode Control/Subsystem2 ==
  x : Inport
  Multiply : Gain  Gain=-1
  Subsystem : Subsystem
  Subsystem1 : Subsystem
  Sum1 : Sum  Inputs=|+-
  sign_x : Outport
  wires:
  Multiply/1 -> Subsystem1/1(In1)
  Subsystem/1(Out1) -> Sum1/1
  Sum1/1 -> sign_x/1
  Subsystem1/1(Out1) -> Sum1/2
  x/1 -> Subsystem/1(In1), Multiply/1

== system Teleoperation_Config_Space/Slave controller/Subsystem1/Subsystem2/Subsystem ==
  In1 : Inport
  Abs1 : Abs
  Constant : Constant
  Divide : Product  Inputs=*/
  Floor1 : Rounding
  Sum1 : Sum  Inputs=|++
  Out1 : Outport
  wires:
  Divide/1 -> Floor1/1
  Constant/1 -> Sum1/2
  Abs1/1 -> Sum1/1
  In1/1 -> Abs1/1, Divide/1
  Sum1/1 -> Divide/2
  Floor1/1 -> Out1/1

== system Teleoperation_Config_Space/Slave controller/Subsystem1/Subsystem2/Subsystem1 ==
  In1 : Inport
  Abs1 : Abs
  Constant : Constant
  Divide : Product  Inputs=*/
  Floor1 : Rounding
  Sum1 : Sum  Inputs=|++
  Out1 : Outport
  wires:
  Divide/1 -> Floor1/1
  Constant/1 -> Sum1/2
  Abs1/1 -> Sum1/1
  In1/1 -> Abs1/1, Divide/1
  Sum1/1 -> Divide/2
  Floor1/1 -> Out1/1

== system Teleoperation_Config_Space/UR5 Master Observer and Force Estimator/Sliding Mode Control/Subsystem2/Subsystem ==
  In1 : Inport
  Abs1 : Abs
  Constant : Constant
  Divide : Product  Inputs=*/
  Floor1 : Rounding
  Sum1 : Sum  Inputs=|++
  Out1 : Outport
  wires:
  Divide/1 -> Floor1/1
  Constant/1 -> Sum1/2
  Abs1/1 -> Sum1/1
  In1/1 -> Abs1/1, Divide/1
  Sum1/1 -> Divide/2
  Floor1/1 -> Out1/1

== system Teleoperation_Config_Space/UR5 Master Observer and Force Estimator/Sliding Mode Control/Subsystem2/Subsystem1 ==
  In1 : Inport
  Abs1 : Abs
  Constant : Constant
  Divide : Product  Inputs=*/
  Floor1 : Rounding
  Sum1 : Sum  Inputs=|++
  Out1 : Outport
  wires:
  Divide/1 -> Floor1/1
  Constant/1 -> Sum1/2
  Abs1/1 -> Sum1/1
  In1/1 -> Abs1/1, Divide/1
  Sum1/1 -> Divide/2
  Floor1/1 -> Out1/1

== system Teleoperation_Config_Space/UR5 Slave Observer and Force Estimator/Sliding Mode Control/Subsystem2/Subsystem ==
  In1 : Inport
  Abs1 : Abs
  Constant : Constant
  Divide : Product  Inputs=*/
  Floor1 : Rounding
  Sum1 : Sum  Inputs=|++
  Out1 : Outport
  wires:
  Divide/1 -> Floor1/1
  Constant/1 -> Sum1/2
  Abs1/1 -> Sum1/1
  In1/1 -> Abs1/1, Divide/1
  Sum1/1 -> Divide/2
  Floor1/1 -> Out1/1

== system Teleoperation_Config_Space/UR5 Slave Observer and Force Estimator/Sliding Mode Control/Subsystem2/Subsystem1 ==
  In1 : Inport
  Abs1 : Abs
  Constant : Constant
  Divide : Product  Inputs=*/
  Floor1 : Rounding
  Sum1 : Sum  Inputs=|++
  Out1 : Outport
  wires:
  Divide/1 -> Floor1/1
  Constant/1 -> Sum1/2
  Abs1/1 -> Sum1/1
  In1/1 -> Abs1/1, Divide/1
  Sum1/1 -> Divide/2
  Floor1/1 -> Out1/1

== matlab function Teleoperation_Config_Space/UR5 Master Observer and Force Estimator/MATLAB Function1 ==
  data: B output; q input; dh parameter
function B = B_q(q, dh)
     B = B_rne(dh, q);

== matlab function Teleoperation_Config_Space/J/MATLAB Function ==
  data: J output; q input; dh parameter
function J = J_q(q, dh)
    J = pinv(J_rne(dh, q)');

== matlab function Teleoperation_Config_Space/UR5 Master Observer and Force Estimator/Estimated Robot Model/MATLAB Function2 ==
  data ddq_ settings: updateMethod=SF_CONTINUOUS_TIME_DATA
  data dq_ settings: updateMethod=SF_CONTINUOUS_TIME_DATA
  data dq settings: updateMethod=SF_CONTINUOUS_TIME_DATA
  data q settings: updateMethod=SF_CONTINUOUS_TIME_DATA
  data u settings: updateMethod=SF_CONTINUOUS_TIME_DATA
  data: ddq_ output size=dh.dof; dq_ output; dq input size=dh.dof; q input size=dh.dof; u input size=dh.dof; g input size=3; dh parameter
function [ddq_, dq_]  = RobotSystem(dq, q, u, g, dh)
    
    % compute dynamics
    B = B_rne(dh, q);
    C = C_rne(dh, q, dq);
    G = G_rne(dh, q, g);
    
    dq_ = dq(1:6);

    ddq = B \ (u - C*dq - G);
    ddq_ = ddq(1:6);

== matlab function Teleoperation_Config_Space/Master/MATLAB Function ==
  data: dq output; q input; dq input; u input; UR5_robot parameter; ddq output
function [dq, ddq] = RobotModel(q, dq, u, UR5_robot)
    B = massMatrix(UR5_robot, q);
    Cdq = velocityProduct(UR5_robot, q, dq);
    G = gravityTorque(UR5_robot, q);
    
    ddq = B \ (u - Cdq - G);
end

== matlab function Teleoperation_Config_Space/Master Controller/Master Controller ==
  data: dh parameter; q input; Fm output; dq input; Fh input; Fe_d input; gravity parameter; qd input; M_m parameter; B_m parameter; K_m parameter
function Fm = Cm(dh,q,dq, Fh,Fe_d,gravity, qd, M_m,B_m,K_m)

    B = B_rne(dh, q);
    C = C_rne(dh, q, dq);
    G = G_rne(dh, q, gravity);
    

    % inner impedance controller
    vm = M_m \ (-B_m*dq - K_m*(q - qd) + Fh - Fe_d);
    % outer decoupling/linearization controller
    Fm = B*vm + C*dq + G - Fh;

== matlab function Teleoperation_Config_Space/Master1/MATLAB Function ==
  data: dX output; X input; dX input; qprev input; u input; UR5_robot parameter; ddX output
function [dX, ddX] = RobotModel(X, dX, qprev, u, UR5_robot)
    
    IK = inverseKinematics();
    q = IK('ee_link', X, [1 1 1 1 1 1], qprev);
    J = geometricJacobian(UR5_robot,q,'ee_link');
    J = [J(4:6,:); J(1:3,:)];
    JD = [];
    Ta = TA(X);
    JA = Ta\J;
    dq = pinv(JA) * dX;
    
    B = massMatrix(UR5_robot, q);
    Cdq = velocityProduct(UR5_robot, q, dq);
    G = gravityTorque(UR5_robot, q);

    BA = inv(JA/B*JA');
    CAdX = BA*(JA/B*C*dq - Ta\(JD*dq - TAD*JA*dq));
    
    ddX = B \ (u - Cdq - G);
end

== matlab function Teleoperation_Config_Space/UR5 Slave/JT/MATLAB Function ==
  data: JT output; q input; dh parameter
function JT = JT_q(q, dh)
    JT = J_rne(dh, q)';

== matlab function Teleoperation_Config_Space/UR5 Slave/Robot Model/MATLAB Function ==
  data ddq_ settings: updateMethod=SF_CONTINUOUS_TIME_DATA
  data dq_ settings: updateMethod=SF_CONTINUOUS_TIME_DATA
  data dq settings: updateMethod=SF_CONTINUOUS_TIME_DATA
  data q settings: updateMethod=SF_CONTINUOUS_TIME_DATA
  data u settings: updateMethod=SF_CONTINUOUS_TIME_DATA
  data: ddq_ output size=dh.dof; dq_ output; dq input size=dh.dof; q input size=dh.dof; u input size=dh.dof; g input size=3; dh parameter
function [ddq_, dq_]  = RobotSystem(dq, q, u, g, dh)
    
    % compute dynamics
    B = B_rne(dh, q);
    C = C_rne(dh, q, dq);
    G = G_rne(dh, q, g);

    dq_ = dq(1:6);

    ddq = B \ (u - C*dq - G);
    ddq_ = ddq(1:6);

== matlab function Teleoperation_Config_Space/UR5 Slave Observer and Force Estimator/Estimated Robot Model/MATLAB Function2 ==
  data ddq_ settings: updateMethod=SF_CONTINUOUS_TIME_DATA
  data dq_ settings: updateMethod=SF_CONTINUOUS_TIME_DATA
  data dq settings: updateMethod=SF_CONTINUOUS_TIME_DATA
  data q settings: updateMethod=SF_CONTINUOUS_TIME_DATA
  data u settings: updateMethod=SF_CONTINUOUS_TIME_DATA
  data: ddq_ output size=dh.dof; dq_ output; dq input size=dh.dof; q input size=dh.dof; u input size=dh.dof; g input size=3; dh parameter
function [ddq_, dq_]  = RobotSystem(dq, q, u, g, dh)
    
    % compute dynamics
    B = B_rne(dh, q);
    C = C_rne(dh, q, dq);
    G = G_rne(dh, q, g);
    
    dq_ = dq(1:6);

    ddq = B \ (u - C*dq - G);
    ddq_ = ddq(1:6);

== matlab function Teleoperation_Config_Space/UR5 Slave Observer and Force Estimator/MATLAB Function1 ==
  data: B output; q input; dh parameter
function B = B_q(q, dh)
     B = B_rne(dh, q);
end

== matlab function Teleoperation_Config_Space/Slave controller/Slave Controller ==
  data: dh parameter; gravity parameter; q_s input; Fs output; dq_s input; q_m input; dq_m input; Fh input; Fe input; Fedd input; qd input; zdq_eq_s input; zdq_eq_m input; sign_s input; M_m parameter; B_m parameter; K_m parameter; M_s parameter; B_s parameter; K_s parameter; K_g parameter
function Fs = Cs(dh,gravity, q_s,dq_s, q_m,dq_m, Fh,Fe,Fedd, qd, zdq_eq_s,zdq_eq_m,sign_s, M_m,B_m,K_m, M_s,B_s,K_s,K_g)

    Ms = B_rne(dh, q_s);
    Cs = C_rne(dh, q_s, dq_s);
    Gs = G_rne(dh, q_s, gravity);
    hs = Cs*dq_s + Gs;

    % TODO needs the master dh, but in this project we have the same robots
    Mm = B_rne(dh, q_m);
    
    Fs = -Ms * (M_s\K_s*(q_s - qd) + M_s\B_s*dq_s ...
                - Ms\hs ...
                + (M_m\K_m - M_s\K_s)*(q_m - qd) ...
                + (M_m\B_m - M_s\B_s)*dq_m ...
                - (inv(M_m) - inv(Mm))*Fh ...
                + M_m\Fedd + M_s\Fe ...
                + zdq_eq_s + zdq_eq_m + K_g*sign_s);

== matlab function Teleoperation_Config_Space/UR5 Master/JT/MATLAB Function ==
  data: JT output; q input; dh parameter
function JT = JT_q(q, dh)
    JT = J_rne(dh, q)';

== matlab function Teleoperation_Config_Space/UR5 Master/Robot Model/MATLAB Function ==
  data ddq_ settings: updateMethod=SF_CONTINUOUS_TIME_DATA
  data dq_ settings: updateMethod=SF_CONTINUOUS_TIME_DATA
  data dq settings: updateMethod=SF_CONTINUOUS_TIME_DATA
  data q settings: updateMethod=SF_CONTINUOUS_TIME_DATA
  data u settings: updateMethod=SF_CONTINUOUS_TIME_DATA
  data: ddq_ output size=dh.dof; dq_ output; dq input size=dh.dof; q input size=dh.dof; u input size=dh.dof; g input size=3; dh parameter
function [ddq_, dq_]  = RobotSystem(dq, q, u, g, dh)
    
    % compute dynamics
    B = B_rne(dh, q);
    C = C_rne(dh, q, dq);
    G = G_rne(dh, q, g);

    dq_ = dq(1:6);

    ddq = B \ (u - C*dq - G);
    ddq_ = ddq(1:6);
